simulink model "kinematics_practice5_2024b"  (R2024b)
settings: Solver=VariableStepAuto  StartTime=0.0  StopTime=2  RelTol=1e-3
InitFcn:
  | %% environmental parameter
  | 
  | g = 9.81;                       %[m/ss]
  | 
  | %% Vehicle parameter
  | 
  | mass = 1.5;                     %[kg]
  | Arm_Length = 0.225;             %[m]
  | 
  | %% Motor parameter
  | 
  | rad2rpm = 60 / (2 * pi);
  | 
  | rpm2rad = 1 / rad2rpm;
  | 
  | Friction_Coef = 0.0001;         %[N m /s]
  | 
  | Inertia = 2.8e-05;              %[kg m^2]
  | 
  | Resistance = 0.1170;            %[ohm]
  | 
  | K_Torque = 1 / (rpm2rad * 960); %[N m/A]
  | 
  | K_Emf = K_Torque;               %[V s/rad]
  | 
  | Tau = (Inertia * Resistance) / (Resistance * Friction_Coef + K_Torque + K_Emf);
  | 
  | ks = K_Torque / (Resistance * Friction_Coef + K_Torque * K_Emf);
  | 
  | Thrust_Coef = 1.1768e-05;
  | 
  | Drag_Coef = 1.8542e-07;
  | 
  | Hovering_Motor_Speed = sqrt(mass * g / (4 * Thrust_Coef));
settings Model: Creator=user  LastModifiedBy=user

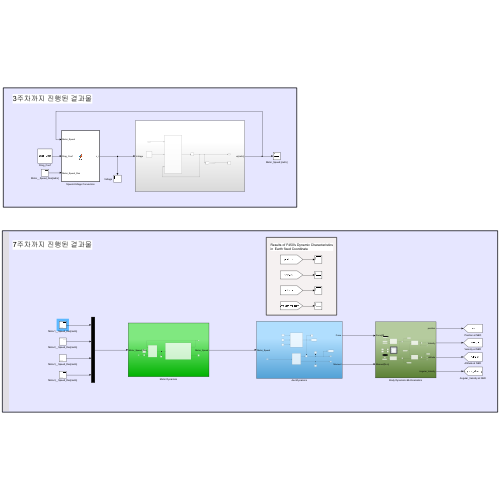
[thumbnail: Simulink's stored preview of the top-level diagram]
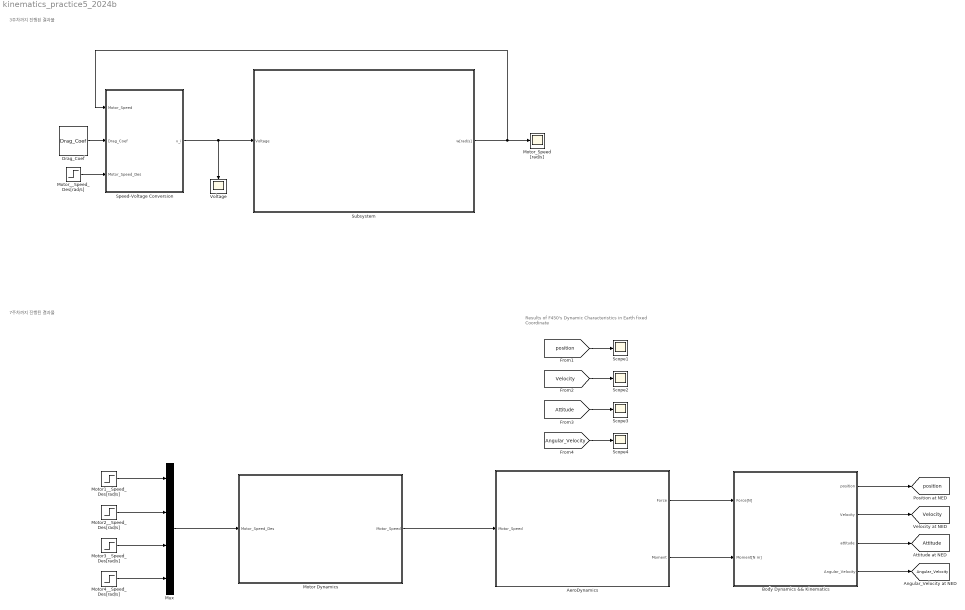
== system kinematics_practice5_2024b ==
  note: Results of F450's Dynamic Characteristics
      | in Earth fixed Coordinate
  note: 3주차까지 진행된 결과물
  note: 7주차까지 진행된 결과물
  AeroDynamics : Subsystem
  Body Dynamics && Kinematics : Subsystem
  Drag_Coef : Constant  Value=Drag_Coef
  Motor Dynamics : Subsystem
  Motor1__Speed_Des[rad/s] : Step  After=Hovering_Motor_Speed  SampleTime=0
  Motor2__Speed_Des[rad/s] : Step  After=Hovering_Motor_Speed  SampleTime=0
  Motor3__Speed_Des[rad/s] : Step  After=Hovering_Motor_Speed  SampleTime=0
  Motor4__Speed_Des[rad/s] : Step  After=Hovering_Motor_Speed  SampleTime=0
  Motor_Speed [rad/s] : Scope
  Motor__Speed_Des[rad/s] : Step  After=Hovering_Motor_Speed  SampleTime=0
  Mux : Mux
  Scope{1..4} (4 alike) : Scope
  Speed-Voltage Conversion : MATLAB Function  TreatAsAtomicUnit=on
  Subsystem : Subsystem
  Voltage : Scope
  tag scope: Angular_Velocity=global, Attitude=global, Velocity=global, position=global
  wires:
  Motor1__Speed_Des[rad/s]/1 -> Mux/1
  Motor2__Speed_Des[rad/s]/1 -> Mux/2
  Motor3__Speed_Des[rad/s]/1 -> Mux/3
  Motor4__Speed_Des[rad/s]/1 -> Mux/4
  Mux/1 -> Motor Dynamics/1(Motor_Speed_Des)
  Motor Dynamics/1(Motor_Speed) -> AeroDynamics/1(Motor_Speed)
  Motor__Speed_Des[rad/s]/1 -> Speed-Voltage Conversion/3(Motor_Speed_Des)
  Speed-Voltage Conversion/1(v_i) -> Voltage/1, Subsystem/1(Voltage)
  Drag_Coef/1 -> Speed-Voltage Conversion/2(Drag_Coef)
  Subsystem/1(w[rad/s]) -> Speed-Voltage Conversion/1(Motor_Speed), Motor_Speed [rad/s]/1
  Body Dynamics && Kinematics/3(attitude) -> [Attitude]
  Body Dynamics && Kinematics/1(position) -> [position]
  [Velocity] -> Scope2/1
  [position] -> Scope1/1
  AeroDynamics/1(Force) -> Body Dynamics && Kinematics/1(Force[N])
  AeroDynamics/2(Moment) -> Body Dynamics && Kinematics/2(Moment[N m])
  Body Dynamics && Kinematics/2(Velocity) -> [Velocity]
  Body Dynamics && Kinematics/4(Angular_Velocity) -> [Angular_Velocity]
  [Attitude] -> Scope3/1
  [Angular_Velocity] -> Scope4/1

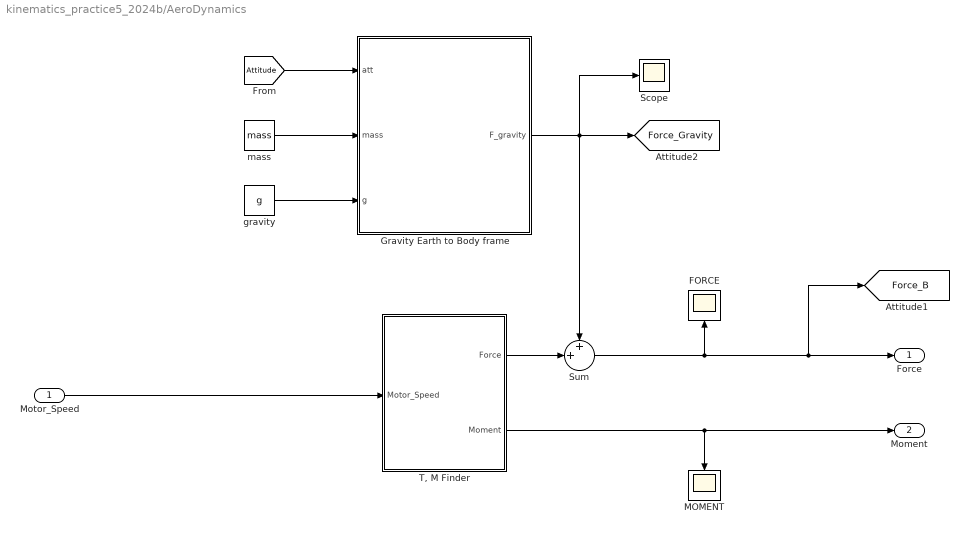
== system kinematics_practice5_2024b/AeroDynamics ==
  Motor_Speed : Inport
  FORCE : Scope
  Gravity Earth to Body frame : MATLAB Function  TreatAsAtomicUnit=on
  MOMENT : Scope
  Scope : Scope
  Sum : Sum  Inputs=++|
  "T, M Finder" : MATLAB Function  TreatAsAtomicUnit=on
  gravity : Constant  Value=g
  mass : Constant  Value=mass
  Force : Outport
  Moment : Outport  Port=2
  tag scope: Force_B=global, Force_Gravity=global
  wires:
  [Attitude] -> Gravity Earth to Body frame/1(att)
  Gravity Earth to Body frame/1(F_gravity) -> Scope/1, [Force_Gravity], Sum/1
  Motor_Speed/1 -> "T, M Finder"/1(Motor_Speed)
  mass/1 -> Gravity Earth to Body frame/2(mass)
  "T, M Finder"/1(Force) -> Sum/2
  gravity/1 -> Gravity Earth to Body frame/3(g)
  Sum/1 -> [Force_B], Force/1, FORCE/1
  "T, M Finder"/2(Moment) -> Moment/1, MOMENT/1

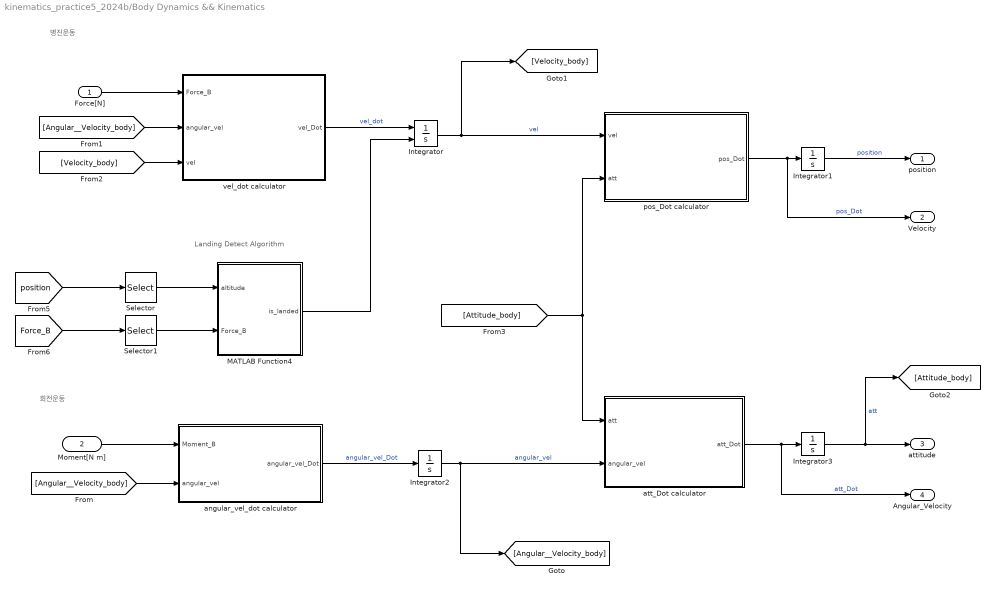
== system kinematics_practice5_2024b/Body Dynamics && Kinematics ==
  note: Landing Detect Algorithm
  note: 병진운동
  note: 회전운동
  Force[N] : Inport
  Moment[N m] : Inport  Port=2
  Integrator : Integrator  ExternalReset=level hold  InitialCondition=[0 0 0]'
  Integrator1 : Integrator  InitialCondition=[0 0 0]'  LimitOutput=on  UpperSaturationLimit=[inf inf 0]'  LowerSaturationLimit=[-inf -inf -inf]'  ZeroCross=off
  Integrator2 : Integrator  InitialCondition=[0 0 0]'
  Integrator3 : Integrator  InitialCondition=[0 0 0]'  WrapState=on
  MATLAB Function4 : MATLAB Function  TreatAsAtomicUnit=on
  Selector : Selector  InputPortWidth=3  IndexOptions=Index vector (dialog)  Indices=[3]  OutputSizes=1
  Selector1 : Selector  InputPortWidth=3  IndexOptions=Index vector (dialog)  Indices=[3]  OutputSizes=1
  angular_vel_dot calculator : MATLAB Function  TreatAsAtomicUnit=on
  att_Dot calculator : MATLAB Function  TreatAsAtomicUnit=on
  pos_Dot calculator : MATLAB Function  TreatAsAtomicUnit=on
  vel_dot calculator : MATLAB Function  TreatAsAtomicUnit=on
  position : Outport
  Velocity : Outport  Port=2
  attitude : Outport  Port=3
  Angular_Velocity : Outport  Port=4
  wires:
  Force[N]/1 -> vel_dot calculator/1(Force_B)
  Moment[N m]/1 -> angular_vel_dot calculator/1(Moment_B)
  Integrator/1 -> pos_Dot calculator/1(vel), [Velocity_body]  "vel"
  pos_Dot calculator/1(pos_Dot) -> Velocity/1, Integrator1/1  "pos_Dot"
  Integrator1/1 -> position/1  "position"
  Integrator2/1 -> att_Dot calculator/2(angular_vel), [Angular__Velocity_body]  "angular_vel"
  Integrator3/1 -> attitude/1, [Attitude_body]  "att"
  att_Dot calculator/1(att_Dot) -> Angular_Velocity/1, Integrator3/1  "att_Dot"
  [Angular__Velocity_body] -> angular_vel_dot calculator/2(angular_vel)
  [Angular__Velocity_body] -> vel_dot calculator/2(angular_vel)
  [Velocity_body] -> vel_dot calculator/3(vel)
  [Attitude_body] -> pos_Dot calculator/2(att), att_Dot calculator/1(att)
  [position] -> Selector/1
  [Force_B] -> Selector1/1
  MATLAB Function4/1(is_landed) -> Integrator/2
  Selector/1 -> MATLAB Function4/1(altitude)
  Selector1/1 -> MATLAB Function4/2(Force_B)
  angular_vel_dot calculator/1(angular_vel_Dot) -> Integrator2/1  "angular_vel_Dot"
  vel_dot calculator/1(vel_Dot) -> Integrator/1  "vel_dot"

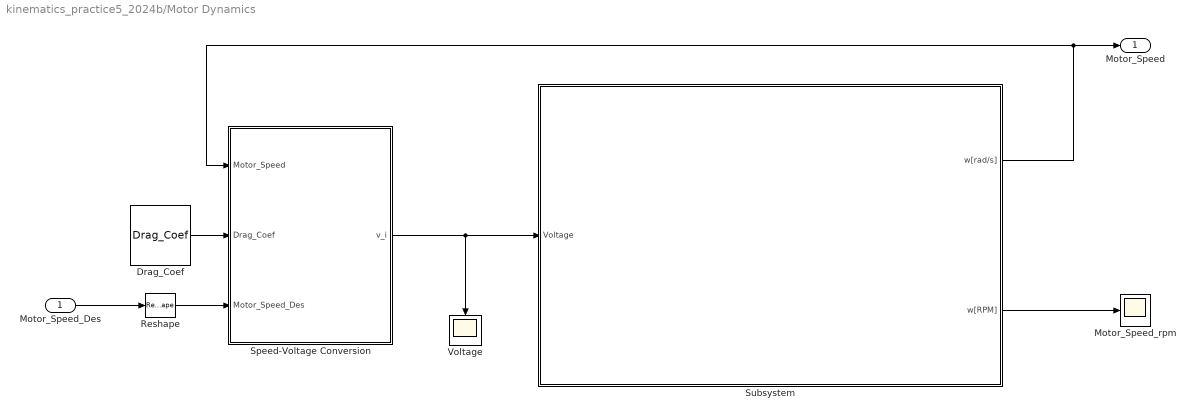
== system kinematics_practice5_2024b/Motor Dynamics ==
  Motor_Speed_Des : Inport
  Drag_Coef : Constant  Value=Drag_Coef
  Motor_Speed_rpm : Scope
  Reshape : Reshape  OutputDimensionality=Column vector (2-D)
  Speed-Voltage Conversion : MATLAB Function  TreatAsAtomicUnit=on
  Subsystem : Subsystem
  Voltage : Scope
  Motor_Speed : Outport
  wires:
  Speed-Voltage Conversion/1(v_i) -> Voltage/1, Subsystem/1(Voltage)
  Drag_Coef/1 -> Speed-Voltage Conversion/2(Drag_Coef)
  Subsystem/1(w[rad/s]) -> Motor_Speed/1, Speed-Voltage Conversion/1(Motor_Speed)
  Subsystem/2(w[RPM]) -> Motor_Speed_rpm/1
  Motor_Speed_Des/1 -> Reshape/1
  Reshape/1 -> Speed-Voltage Conversion/3(Motor_Speed_Des)

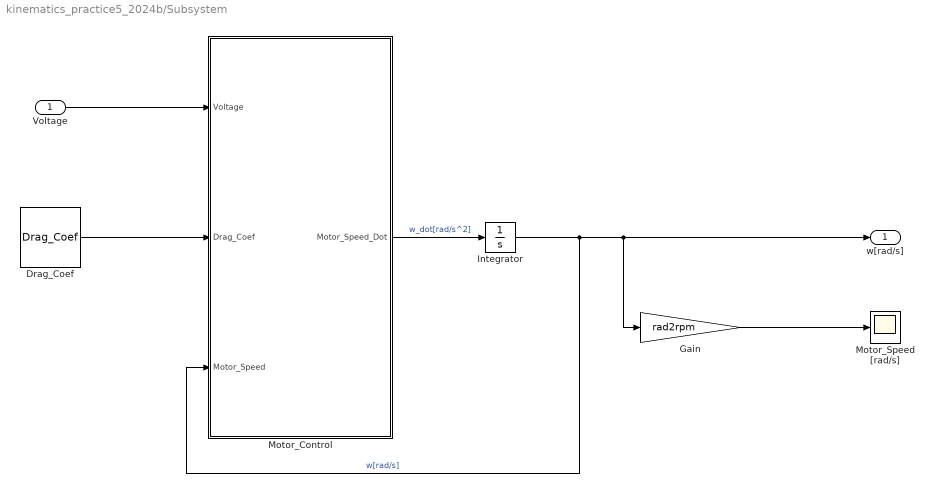
== system kinematics_practice5_2024b/Subsystem ==
  Voltage : Inport
  Drag_Coef : Constant  Value=Drag_Coef
  Gain : Gain  Gain=rad2rpm
  Integrator : Integrator
  Motor_Control : MATLAB Function  TreatAsAtomicUnit=on
  Motor_Speed [rad/s] : Scope
  w[rad/s] : Outport
  wires:
  Motor_Control/1(Motor_Speed_Dot) -> Integrator/1  "w_dot[rad/s^2]"
  Integrator/1 -> w[rad/s]/1, Gain/1, Motor_Control/3(Motor_Speed)  "w[rad/s]"
  Gain/1 -> Motor_Speed [rad/s]/1
  Voltage/1 -> Motor_Control/1(Voltage)
  Drag_Coef/1 -> Motor_Control/2(Drag_Coef)

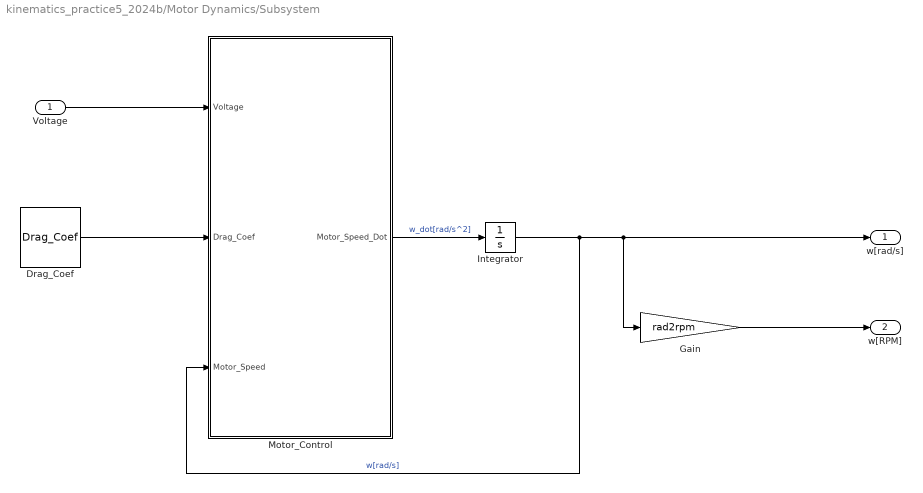
== system kinematics_practice5_2024b/Motor Dynamics/Subsystem ==
  Voltage : Inport
  Drag_Coef : Constant  Value=Drag_Coef
  Gain : Gain  Gain=rad2rpm
  Integrator : Integrator  InitialCondition=[0 0 0 0]'
  Motor_Control : MATLAB Function  TreatAsAtomicUnit=on
  w[rad/s] : Outport
  w[RPM] : Outport  Port=2
  wires:
  Motor_Control/1(Motor_Speed_Dot) -> Integrator/1  "w_dot[rad/s^2]"
  Integrator/1 -> w[rad/s]/1, Gain/1, Motor_Control/3(Motor_Speed)  "w[rad/s]"
  Gain/1 -> w[RPM]/1
  Voltage/1 -> Motor_Control/1(Voltage)
  Drag_Coef/1 -> Motor_Control/2(Drag_Coef)

== matlab function kinematics_practice5_2024b/Body Dynamics && Kinematics/MATLAB Function4 ==
  data: is_landed output; altitude input; Force_B input
function is_landed = fcn(altitude, Force_B)

is_landed = (altitude >= 0) && (Force_B > 0);

end

== matlab function kinematics_practice5_2024b/Motor Dynamics/Speed-Voltage Conversion ==
  data: Motor_Speed input; Drag_Coef input; Motor_Speed_Des input; v_i output
function v_i = fcn(Motor_Speed, Drag_Coef, Motor_Speed_Des)

rad2rpm = 60 / (2 * pi);

rpm2rad = 1 / rad2rpm;

Resistance = 0.1170;            %[ohm]

K_Torque = 1 / (rpm2rad * 960); %[N m/A]

K_Emf = K_Torque;               %[V s/rad]


v_i = K_Emf .* Motor_Speed_Des + Resistance/K_Torque * Drag_Coef .* Motor_Speed.^2;


end

== matlab function kinematics_practice5_2024b/Motor Dynamics/Subsystem/Motor_Control ==
  data: Voltage input; Drag_Coef input; Motor_Speed_Dot output; Motor_Speed input
function Motor_Speed_Dot = fcn(Voltage, Drag_Coef, Motor_Speed)

rad2rpm = 60 / (2 * pi);

rpm2rad = 1 / rad2rpm;

Inertia = 2.8e-05;              %[kg m^2]

Resistance = 0.1170;            %[ohm]

K_Torque = 1 / (rpm2rad * 960); %[N m/A]

K_Emf = K_Torque;               %[V s/rad]

V_Emf = K_Emf .* Motor_Speed; %[Voltage]

Current = (Voltage - V_Emf) / Resistance; %[A]

Motor_Speed_Dot = (K_Torque * Current - Drag_Coef * Motor_Speed.^2)/ Inertia; %[rad/s^2]

end

== matlab function kinematics_practice5_2024b/AeroDynamics/T, M Finder ==
  data: Motor_Speed input; Force output; Moment output
function [Force, Moment] = fcn(Motor_Speed)

Thrust_Coef = 1.1768e-05;

Drag_Coef = 1.8542e-07;

Arm_Length = 0.225;             %[m]


Force = [0;
         0;
         -Thrust_Coef * sum(Motor_Speed.^2)];


Drag = Drag_Coef * Motor_Speed.^2; %4x1 matrix, [d] .* [w^2]


Moment = [Arm_Length * Thrust_Coef * (Motor_Speed(4)^2 - Motor_Speed(2)^2);
          Arm_Length * Thrust_Coef * (Motor_Speed(1)^2 - Motor_Speed(3)^2);
          -Drag(1) + Drag(2) - Drag(3) + Drag(4)];

== matlab function kinematics_practice5_2024b/Speed-Voltage Conversion ==
  data: Motor_Speed input; Drag_Coef input; Motor_Speed_Des input; v_i output
function v_i = fcn(Motor_Speed, Drag_Coef, Motor_Speed_Des)

rad2rpm = 60 / (2 * pi);

rpm2rad = 1 / rad2rpm;

Resistance = 0.1170;            %[ohm]

K_Torque = 1 / (rpm2rad * 960); %[N m/A]

K_Emf = K_Torque;               %[V s/rad]


v_i = K_Emf * Motor_Speed_Des + Resistance/K_Torque * Drag_Coef * Motor_Speed^2;


end

== matlab function kinematics_practice5_2024b/Subsystem/Motor_Control ==
  data: Voltage input; Drag_Coef input; Motor_Speed_Dot output; Motor_Speed input
function Motor_Speed_Dot = fcn(Voltage, Drag_Coef, Motor_Speed)

rad2rpm = 60 / (2 * pi);

rpm2rad = 1 / rad2rpm;

Inertia = 2.8e-05;              %[kg m^2]

Resistance = 0.1170;            %[ohm]

K_Torque = 1 / (rpm2rad * 960); %[N m/A]

K_Emf = K_Torque;               %[V s/rad]

V_Emf = K_Emf * Motor_Speed; %[Voltage]

Current = (Voltage - V_Emf) / Resistance; %[A]

Motor_Speed_Dot = (K_Torque * Current - Drag_Coef * Motor_Speed^2)/ Inertia; %[rad/s^2]

end

== matlab function kinematics_practice5_2024b/AeroDynamics/Gravity Earth to Body frame ==
  data: att input; F_gravity output; mass input; g input
function F_gravity = fcn(att, mass, g)

phi = att(1);
theta = att(2);

gravity = g * [-sind(theta);
                sind(phi)*cosd(theta);
                cosd(phi)*cosd(theta)];

F_gravity = mass * gravity;

== matlab function kinematics_practice5_2024b/Body Dynamics && Kinematics/vel_dot calculator ==
  data: Force_B input; vel_Dot output; angular_vel input; vel input
function vel_Dot = fcn(Force_B, angular_vel, vel)
mass = 1.5;
vel_Dot = Force_B / mass - cross(angular_vel, vel);

== matlab function kinematics_practice5_2024b/Body Dynamics && Kinematics/angular_vel_dot calculator ==
  data: Moment_B input; angular_vel_Dot output; angular_vel input
function angular_vel_Dot = fcn(Moment_B, angular_vel)

Inertia = diag([0.02 0.02 0.025]);

angular_vel_Dot = Inertia ^ (-1) * (Moment_B - cross(angular_vel, Inertia * angular_vel));

== matlab function kinematics_practice5_2024b/Body Dynamics && Kinematics/pos_Dot calculator ==
  data: vel input; pos_Dot output; att input
function pos_Dot = fcn(vel, att)
%바디축의 velocity

phi = att(1);
theta = att(2);
psi = att(3);

c_psi = cos(psi);
s_psi = sin(psi);
c_theta = cos(theta);
s_theta = sin(theta);
c_phi = cos(phi);
s_phi = sin(phi);


%R_EB
R_B2E = [c_psi*c_theta      c_psi*s_theta*s_phi-s_psi*c_phi         c_psi*s_theta*c_phi + s_psi*s_phi;
        s_psi*c_theta       s_psi*s_theta*s_phi + c_psi*c_phi       s_psi*s_theta*c_phi - c_psi*s_phi;
           -s_theta                 c_theta*s_phi                               c_theta*c_phi];



pos_Dot = R_B2E * vel;

== matlab function kinematics_practice5_2024b/Body Dynamics && Kinematics/att_Dot calculator ==
  data: att input; angular_vel input; att_Dot output
function att_Dot = fcn(att, angular_vel)

phi = att(1);
theta = att(2);



R_B2E = [1      sin(phi)*tan(theta)     cos(phi)*tan(theta);
         0              cos(phi)            -sin(phi);
         0      sin(phi)*sec(theta)     cos(phi)*sec(theta)];


att_Dot = R_B2E * angular_vel;
